simulink model "CrC_DD"  (R2016b)
settings: configuration reference "CodeGenConfigSet" (kept outside this file)
values from neighbouring files (symbols this model uses):
  CrC_tiMinusDebHiLo_C = Calibration.Parameter    [init_CrC_DD.m]
  CrC_tiMinusDebLoHi_C = Calibration.Parameter    [init_CrC_DD.m]
  CrC_tiOffDebHiLo_C = Calibration.Parameter    [init_CrC_DD.m]
  CrC_tiOffDebLoHi_C = Calibration.Parameter    [init_CrC_DD.m]
  CrC_tiPlusDebHiLo_C = Calibration.Parameter    [init_CrC_DD.m]
  CrC_tiPlusDebLoHi_C = Calibration.Parameter    [init_CrC_DD.m]
  CrC_tiResDebHiLo_C = Calibration.Parameter    [init_CrC_DD.m]
  CrC_tiResDebLoHi_C = Calibration.Parameter    [init_CrC_DD.m]
undefined symbols (not defined in the file or in its folder): CrC_DD_DT
libraries: simulink x8, CXLib x4
settings Model: Creator=xinchangran  LastModifiedBy=xinchangran
settings ConfigSetRef: SourceLocation=Base Workspace

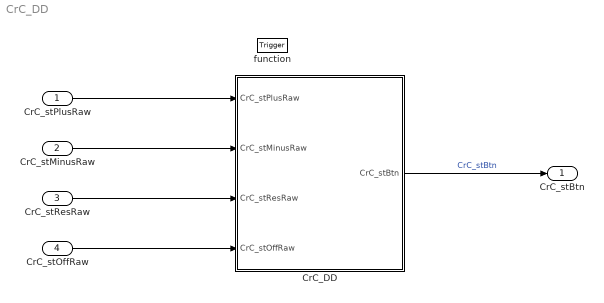
== system CrC_DD ==
  CrC_stPlusRaw : Inport  Description=Plus button  OutMin=0  OutMax=1  OutDataTypeStr=boolean
  CrC_stMinusRaw : Inport  Description=Minus button  Port=2  OutMin=0  OutMax=1  OutDataTypeStr=boolean
  CrC_stResRaw : Inport  Description=Resume button  Port=3  OutMin=0  OutMax=1  OutDataTypeStr=boolean
  CrC_stOffRaw : Inport  Description=Off/On button  Port=4  OutMin=0  OutMax=1  OutDataTypeStr=boolean
  function : TriggerPort  TriggerType=function-call  VariantControl=Variant
  CrC_DD : Subsystem
  CrC_stBtn : Outport  Description=The Cruise control button/0/1/2/3  OutMin=0  OutMax=255  OutDataTypeStr=State_uint8
  wires:
  CrC_stPlusRaw/1 -> CrC_DD/1(CrC_stPlusRaw)
  CrC_stMinusRaw/1 -> CrC_DD/2(CrC_stMinusRaw)
  CrC_stResRaw/1 -> CrC_DD/3(CrC_stResRaw)
  CrC_stOffRaw/1 -> CrC_DD/4(CrC_stOffRaw)
  CrC_DD/1(CrC_stBtn) -> CrC_stBtn/1  "CrC_stBtn"

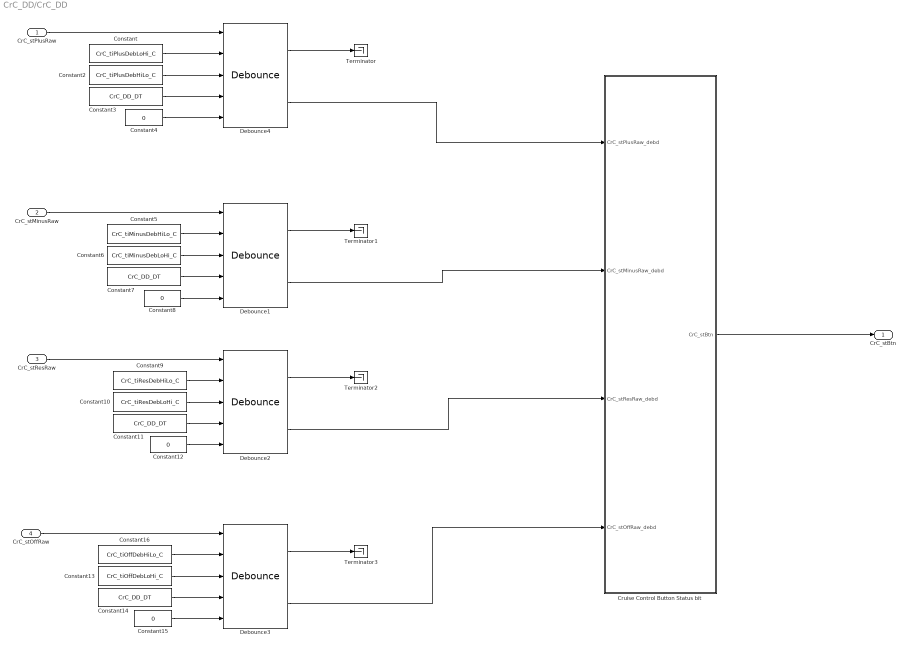
== system CrC_DD/CrC_DD ==
  CrC_stPlusRaw : Inport
  CrC_stMinusRaw : Inport  Port=2
  CrC_stResRaw : Inport  Port=3
  CrC_stOffRaw : Inport  Port=4
  Constant : Constant  Value=CrC_tiPlusDebLoHi_C
  Constant10 : Constant  Value=CrC_tiResDebLoHi_C
  Constant{3,7,11,14} (4 alike) : Constant  Value=CrC_DD_DT
  Constant{4,8,12,15} (4 alike) : Constant  Value=0  OutDataTypeStr=Inherit: Inherit via back propagation
  Constant13 : Constant  Value=CrC_tiOffDebLoHi_C
  Constant16 : Constant  Value=CrC_tiOffDebHiLo_C
  Constant2 : Constant  Value=CrC_tiPlusDebHiLo_C
  Constant5 : Constant  Value=CrC_tiMinusDebHiLo_C
  Constant6 : Constant  Value=CrC_tiMinusDebLoHi_C
  Constant9 : Constant  Value=CrC_tiResDebHiLo_C
  Cruise Control Button Status bit : Subsystem
  Debounce{1..4} (4 alike) : CXLib/Debounce
  Terminator{,1..3} (4 alike) : Terminator
  CrC_stBtn : Outport
  wires:
  Debounce3/1 -> Terminator3/1
  Debounce4/2 -> Cruise Control Button Status bit/1(CrC_stPlusRaw_debd)
  Debounce3/2 -> Cruise Control Button Status bit/4(CrC_stOffRaw_debd)
  Constant3/1 -> Debounce4/4
  Constant2/1 -> Debounce4/3
  Constant4/1 -> Debounce4/5
  Debounce4/1 -> Terminator/1
  Constant/1 -> Debounce4/2
  CrC_stPlusRaw/1 -> Debounce4/1
  Constant10/1 -> Debounce2/3
  Constant9/1 -> Debounce2/2
  Debounce2/1 -> Terminator2/1
  Constant11/1 -> Debounce2/4
  Constant12/1 -> Debounce2/5
  CrC_stOffRaw/1 -> Debounce3/1
  CrC_stMinusRaw/1 -> Debounce1/1
  Constant13/1 -> Debounce3/3
  Constant15/1 -> Debounce3/5
  Constant14/1 -> Debounce3/4
  Constant16/1 -> Debounce3/2
  CrC_stResRaw/1 -> Debounce2/1
  Constant5/1 -> Debounce1/2
  Constant6/1 -> Debounce1/3
  Constant7/1 -> Debounce1/4
  Constant8/1 -> Debounce1/5
  Debounce1/1 -> Terminator1/1
  Debounce1/2 -> Cruise Control Button Status bit/2(CrC_stMinusRaw_debd)
  Cruise Control Button Status bit/1(CrC_stBtn) -> CrC_stBtn/1
  Debounce2/2 -> Cruise Control Button Status bit/3(CrC_stResRaw_debd)

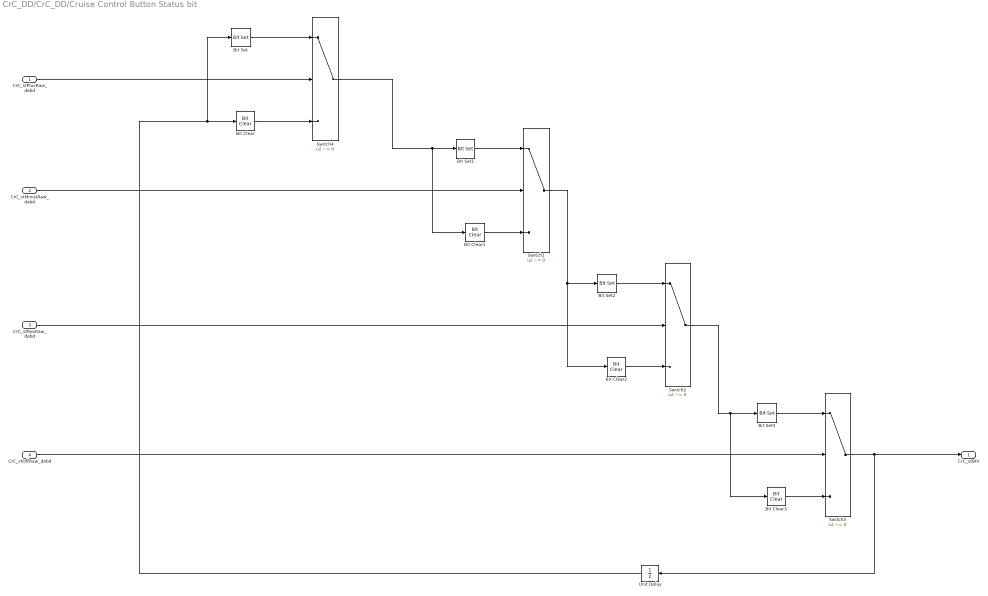
== system CrC_DD/CrC_DD/Cruise Control Button Status bit ==
  CrC_stPlusRaw_debd : Inport
  CrC_stMinusRaw_debd : Inport  Port=2
  CrC_stResRaw_debd : Inport  Port=3
  CrC_stOffRaw_debd : Inport  Port=4
  Bit Clear : simulink/Logic and Bit Operations/Bit Clear  iBit=1
  Bit Clear1 : simulink/Logic and Bit Operations/Bit Clear  iBit=2
  Bit Clear2 : simulink/Logic and Bit Operations/Bit Clear  iBit=3
  Bit Clear3 : simulink/Logic and Bit Operations/Bit Clear  iBit=0
  Bit Set : simulink/Logic and Bit Operations/Bit Set  iBit=1
  Bit Set1 : simulink/Logic and Bit Operations/Bit Set  iBit=2
  Bit Set2 : simulink/Logic and Bit Operations/Bit Set  iBit=3
  Bit Set3 : simulink/Logic and Bit Operations/Bit Set  iBit=0
  Switch{1..4} (4 alike) : Switch  Criteria=u2 ~= 0  InputSameDT=on
  Unit Delay : UnitDelay  SampleTime=-1
      settings: AttributesFormatString=InitialValue=%<InitialCondition>
  CrC_stBtn : Outport
  wires:
  CrC_stPlusRaw_debd/1 -> Switch4/2
  CrC_stMinusRaw_debd/1 -> Switch1/2
  CrC_stResRaw_debd/1 -> Switch2/2
  CrC_stOffRaw_debd/1 -> Switch3/2
  Switch1/1 -> Bit Clear2/1, Bit Set2/1
  Switch2/1 -> Bit Clear3/1, Bit Set3/1
  Bit Set3/1 -> Switch3/1
  Bit Clear3/1 -> Switch3/3
  Bit Clear2/1 -> Switch2/3
  Bit Set2/1 -> Switch2/1
  Bit Clear1/1 -> Switch1/3
  Bit Set1/1 -> Switch1/1
  Bit Set/1 -> Switch4/1
  Bit Clear/1 -> Switch4/3
  Switch4/1 -> Bit Clear1/1, Bit Set1/1
  Switch3/1 -> Unit Delay/1, CrC_stBtn/1
  Unit Delay/1 -> Bit Set/1, Bit Clear/1
